simulink model "simus"  (R2021a)
settings: Solver=VariableStepAuto  StartTime=0.0  StopTime=10  RelTol=1e-3
values from neighbouring files (symbols this model uses):
  A = -Gm.den{1}(end)    [desarrollo.m]
  B = Gm.num{1}(end)    [desarrollo.m]
  C = 1    [desarrollo.m]
  den = Gp.den{1}    [desarrollo.m]
  K = -polyval([den 0],s)/polyval(num,s)    [desarrollo.m]
  K0 = -polyval(den,s)*s/polyval(num,s)    [desarrollo.m]
  K1 = -polyval(den,s)*s/polyval(num,s)    [desarrollo.m]
  Kd = acker(As_d,Bs_d,z)    [desarrollo.m]
  Ki1 = zero*Kp1    [desarrollo.m]
  Kp1 = -(s*polyval(den,s))/polyval(num,s)/(s+zero)    [desarrollo.m]
  num = Gp.num{1}    [desarrollo.m]
  Ts = 4/ro/10    (= 0.0142857142857)    [desarrollo.m]
undefined symbols (not defined in the file or in its folder): DiscIntNeverNeededParam, Gm
settings Model: Creator=pierr  LastModifiedBy=pierr

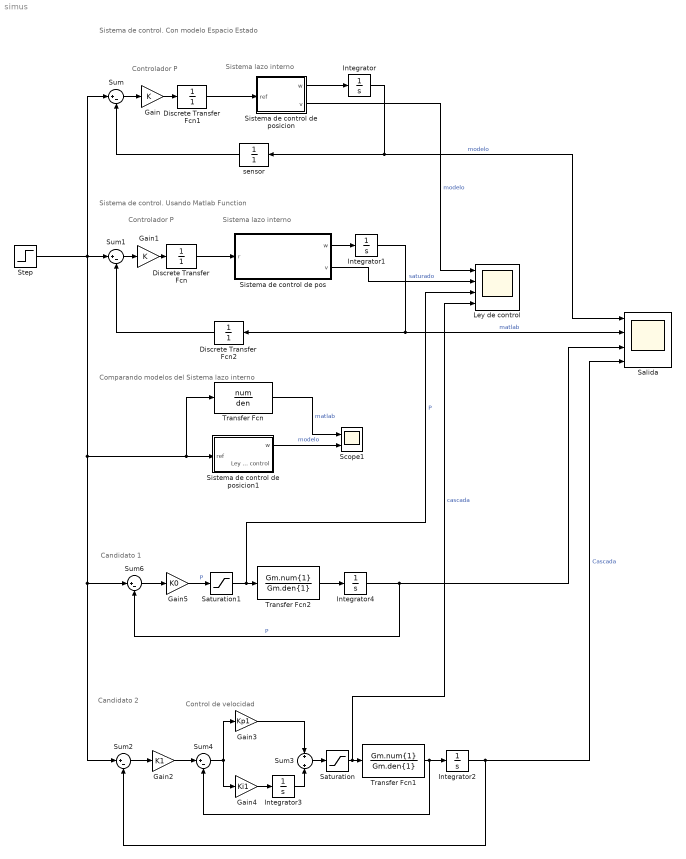
== system simus ==
  note: Comparando modelos del Sistema lazo interno
  note: Sistema lazo interno
  note: Controlador P
  note: Sistema de control. Con modelo Espacio Estado
  note: Sistema lazo interno
  note: Controlador P
  note: Sistema de control. Usando Matlab Function
  note: Candidato 2
  note: Control de velocidad
  note: Candidato 1
  Discrete Transfer Fcn : DiscreteTransferFcn  Denominator=[1]
  Discrete Transfer Fcn1 : DiscreteTransferFcn  Denominator=[1]
  Discrete Transfer Fcn2 : DiscreteTransferFcn  Denominator=[1]
  Gain : Gain  Gain=K
  Gain1 : Gain  Gain=K
  Gain2 : Gain  Gain=K1
  Gain3 : Gain  Gain=Kp1
  Gain4 : Gain  Gain=Ki1
  Gain5 : Gain  Gain=K0
  Integrator{,1..4} (5 alike) : Integrator
  Ley de control : Scope  NumInputPorts=4
  Salida : Scope  NumInputPorts=4
  Saturation : Saturate  UpperLimit=4.8  LowerLimit=-4.8
  Saturation1 : Saturate  UpperLimit=4.8  LowerLimit=-4.8
  Scope1 : Scope  NumInputPorts=2
  Sistema de control de pos : Subsystem
  Sistema de control de posicion : Subsystem
  Sistema de control de posicion1 : Subsystem
  Step : Step  Time=0  After=270  SampleTime=Ts
  Sum{,1..2,4,6} (5 alike) : Sum  Inputs=|+-
  Sum3 : Sum  Inputs=+||+
  Transfer Fcn : TransferFcn  Numerator=num  Denominator=den
  Transfer Fcn1 : TransferFcn  Numerator=Gm.num{1}  Denominator=Gm.den{1}
  Transfer Fcn2 : TransferFcn  Numerator=Gm.num{1}  Denominator=Gm.den{1}
  sensor : DiscreteTransferFcn  Denominator=[1]
  wires:
  Sum/1 -> Gain/1
  Sistema de control de posicion/1(w) -> Integrator/1
  Sum1/1 -> Gain1/1
  Sistema de control de pos/1(w) -> Integrator1/1
  Integrator/1 -> sensor/1, Salida/1  "modelo"
  Integrator1/1 -> Discrete Transfer Fcn2/1, Salida/2  "matlab"
  Transfer Fcn/1 -> Scope1/1  "matlab"
  Gain/1 -> Discrete Transfer Fcn1/1
  Discrete Transfer Fcn1/1 -> Sistema de control de posicion/1(ref)
  Gain1/1 -> Discrete Transfer Fcn/1
  Discrete Transfer Fcn/1 -> Sistema de control de pos/1(r)
  Discrete Transfer Fcn2/1 -> Sum1/2
  sensor/1 -> Sum/2
  Sistema de control de posicion/2(v) -> Ley de control/1  "modelo"
  Sistema de control de pos/2(v) -> Ley de control/2  "saturado"
  Sistema de control de posicion1/1(w) -> Scope1/2  "modelo"
  Saturation/1 -> Ley de control/4, Transfer Fcn1/1  "cascada"
  Transfer Fcn1/1 -> Sum4/2, Integrator2/1
  Integrator2/1 -> Sum2/2, Salida/4  "Cascada"
  Gain2/1 -> Sum4/1
  Step/1 -> Sum6/1, Sum2/1, Transfer Fcn/1, Sistema de control de posicion1/1(ref), Sum/1, Sum1/1
  Sum4/1 -> Gain3/1, Gain4/1
  Integrator3/1 -> Sum3/2
  Gain3/1 -> Sum3/1
  Sum3/1 -> Saturation/1
  Gain4/1 -> Integrator3/1
  Sum2/1 -> Gain2/1
  Gain5/1 -> Saturation1/1  "P"
  Saturation1/1 -> Ley de control/3, Transfer Fcn2/1  "P"
  Transfer Fcn2/1 -> Integrator4/1
  Sum6/1 -> Gain5/1
  Integrator4/1 -> Sum6/2, Salida/3  "P"

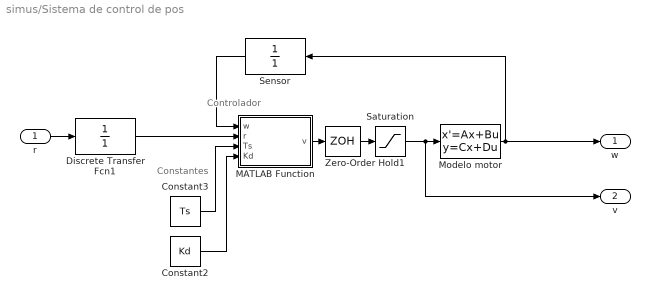
== system simus/Sistema de control de pos ==
  note: Controlador
  note: Constantes
  r : Inport
  Constant2 : Constant  Value=Kd
  Constant3 : Constant  Value=Ts
  Discrete Transfer Fcn1 : DiscreteTransferFcn  Denominator=[1]  SampleTime=Ts
  MATLAB Function : MATLAB Function  TreatAsAtomicUnit=on
  Modelo motor : StateSpace  A=A  B=B  C=C  D=0  InitialCondition=0
  Saturation : Saturate  UpperLimit=5  LowerLimit=-5
  Sensor : DiscreteTransferFcn  Denominator=[1]  SampleTime=Ts
  Zero-Order Hold1 : ZeroOrderHold  SampleTime=Ts
  w : Outport
  v : Outport  Port=2
  wires:
  MATLAB Function/1(v) -> Zero-Order Hold1/1
  Constant3/1 -> MATLAB Function/3(Ts)
  Modelo motor/1 -> w/1, Sensor/1
  Sensor/1 -> MATLAB Function/1(w)
  Constant2/1 -> MATLAB Function/4(Kd)
  r/1 -> Discrete Transfer Fcn1/1
  Discrete Transfer Fcn1/1 -> MATLAB Function/2(r)
  Saturation/1 -> v/1, Modelo motor/1
  Zero-Order Hold1/1 -> Saturation/1

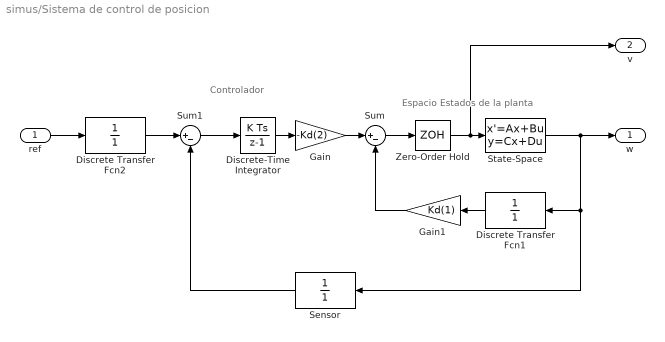
== system simus/Sistema de control de posicion ==
  note: Controlador
  note: Espacio Estados de la planta
  ref : Inport
  Discrete Transfer Fcn1 : DiscreteTransferFcn  Denominator=[1]  SampleTime=Ts
  Discrete Transfer Fcn2 : DiscreteTransferFcn  Denominator=[1]  SampleTime=Ts
  Discrete-Time Integrator : DiscreteIntegrator  SampleTime=Ts  ICPrevOutput=DiscIntNeverNeededParam  ICPrevScaledInput=DiscIntNeverNeededParam
  Gain : Gain  Gain=-Kd(2)
  Gain1 : Gain  Gain=Kd(1)
  Sensor : DiscreteTransferFcn  Denominator=[1]  SampleTime=Ts
  State-Space : StateSpace  A=A  B=B  C=C  D=0  InitialCondition=0
  Sum : Sum  Inputs=|+-
  Sum1 : Sum  Inputs=|+-
  Zero-Order Hold : ZeroOrderHold  SampleTime=Ts
  w : Outport
  v : Outport  Port=2
  wires:
  Sensor/1 -> Sum1/2
  Sum1/1 -> Discrete-Time Integrator/1
  State-Space/1 -> w/1, Sensor/1, Discrete Transfer Fcn1/1
  Discrete-Time Integrator/1 -> Gain/1
  Discrete Transfer Fcn1/1 -> Gain1/1
  Gain/1 -> Sum/1
  Gain1/1 -> Sum/2
  Sum/1 -> Zero-Order Hold/1
  Zero-Order Hold/1 -> v/1, State-Space/1
  ref/1 -> Discrete Transfer Fcn2/1
  Discrete Transfer Fcn2/1 -> Sum1/1

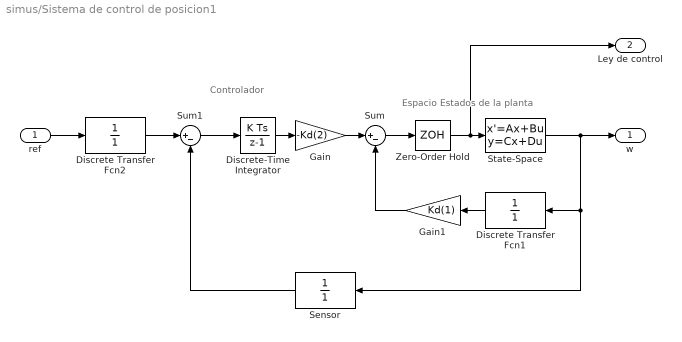
== system simus/Sistema de control de posicion1 ==
  note: Controlador
  note: Espacio Estados de la planta
  ref : Inport
  Discrete Transfer Fcn1 : DiscreteTransferFcn  Denominator=[1]  SampleTime=Ts
  Discrete Transfer Fcn2 : DiscreteTransferFcn  Denominator=[1]  SampleTime=Ts
  Discrete-Time Integrator : DiscreteIntegrator  SampleTime=Ts  ICPrevOutput=DiscIntNeverNeededParam  ICPrevScaledInput=DiscIntNeverNeededParam
  Gain : Gain  Gain=-Kd(2)
  Gain1 : Gain  Gain=Kd(1)
  Sensor : DiscreteTransferFcn  Denominator=[1]  SampleTime=Ts
  State-Space : StateSpace  A=A  B=B  C=C  D=0  InitialCondition=0
  Sum : Sum  Inputs=|+-
  Sum1 : Sum  Inputs=|+-
  Zero-Order Hold : ZeroOrderHold  SampleTime=Ts
  w : Outport
  Ley de control : Outport  Port=2
  wires:
  Sensor/1 -> Sum1/2
  Sum1/1 -> Discrete-Time Integrator/1
  State-Space/1 -> w/1, Sensor/1, Discrete Transfer Fcn1/1
  Discrete-Time Integrator/1 -> Gain/1
  Discrete Transfer Fcn1/1 -> Gain1/1
  Gain/1 -> Sum/1
  Gain1/1 -> Sum/2
  Sum/1 -> Zero-Order Hold/1
  Zero-Order Hold/1 -> Ley de control/1, State-Space/1
  ref/1 -> Discrete Transfer Fcn2/1
  Discrete Transfer Fcn2/1 -> Sum1/1

== matlab function simus/Sistema de control de pos/MATLAB Function ==
  settings: updateMethod=DISCRETE
  data: w input; v output; r input; Ts input; Kd input
function v = fcn(w,r,Ts,Kd)

persistent ek_1
persistent x2_1
if isempty (ek_1)
    ek_1=0;
    x2_1=0;
end
ek=r-w;
x2=x2_1+Ts/2*(ek+ek_1);
v = -Kd(1)*w-Kd(2)*x2;

ek_1=ek;
x2_1=x2;
